simulink model "Half_wave_rectification"  (R2020a)
settings: Solver=VariableStepAuto  StartTime=0.0  StopTime=10.0  RelTol=1e-3
settings Model: Creator=11973  LastModifiedBy=11973

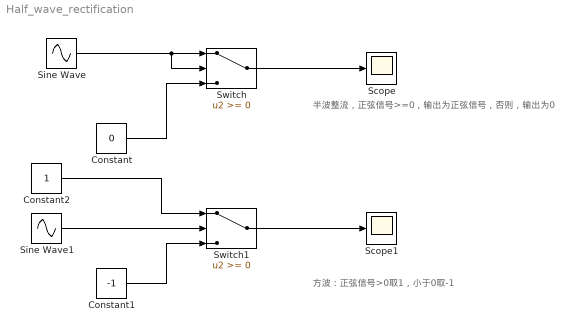
== system Half_wave_rectification ==
  note: 半波整流，正弦信号>=0，输出为正弦信号，否则，输出为0
  note: 方波：正弦信号>0取1，小于0取-1
  Constant : Constant  Value=0
  Constant1 : Constant  Value=-1
  Constant2 : Constant
  Scope : Scope
  Scope1 : Scope
  Sine Wave : Sin  SampleTime=0
  Sine Wave1 : Sin  SampleTime=0
  Switch : Switch
  Switch1 : Switch
  wires:
  Sine Wave/1 -> Switch/2, Switch/1
  Constant/1 -> Switch/3
  Switch/1 -> Scope/1
  Switch1/1 -> Scope1/1
  Constant1/1 -> Switch1/3
  Sine Wave1/1 -> Switch1/2
  Constant2/1 -> Switch1/1
